simulink model "Discret_algemeine_schematische"  (Simulink 7.7)
settings: Solver=ode45  StartTime=0.0  StopTime=14  RelTol=1e-3
libraries: simulink x5
settings Model: Creator=evgenov  LastModifiedBy=Алексей
settings DebuggingCC: FcnCallInpInsideContextMsg=Enable All

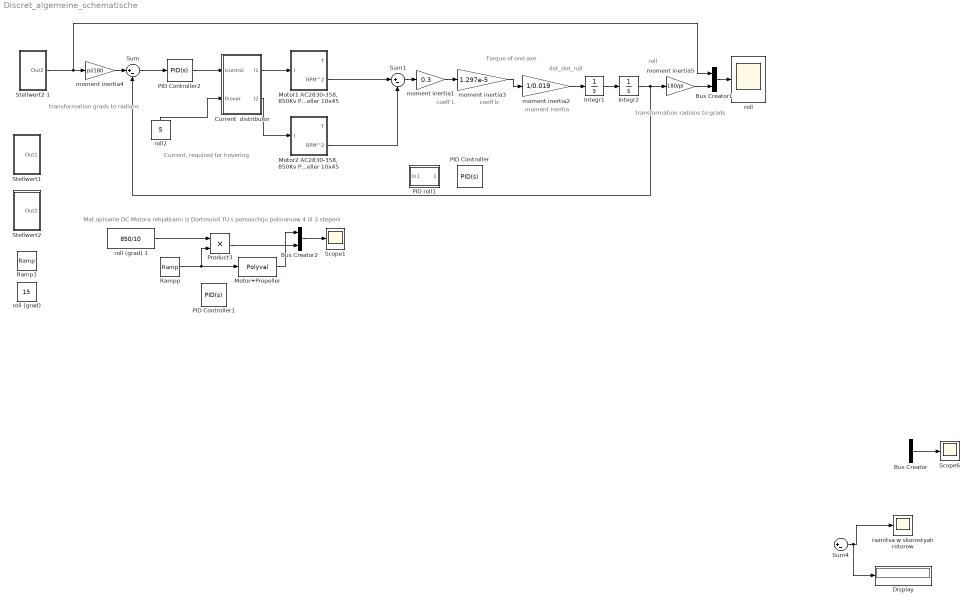
== system Discret_algemeine_schematische ==
  note: roll
  note: dot_dot_roll
  note: moment inertia
  note: Mat.opisanie DC Motora
      | rebjatkami iz Dortmund TU s pomoschiju
      | polinomow 4 ili 3 stepeni
  note: coeff L
  note: coeff b
  note: Torque of
      | one axe
  note: transformation
      | grads to radians
  note: transformation
      | radians to grads
  note: Current, required
      | for hovering
  Bus Creator : BusCreator  Inputs=2
  Bus Creator1 : BusCreator  Inputs=2
  Bus Creator2 : BusCreator  Inputs=2
  Current  distributor : Subsystem
  Display : Display
  Integr1 : Integrator
  Integr2 : Integrator
  Motor+Propeller : Polyval  Coefs="[0.0125   -0.1814   -3.6987  124.7646  -0.0000]"
  "Motor1 AC2830-358,  850Kv Propeller 10x45" : Subsystem
  "Motor2 AC2830-358,  850Kv Propeller 10x45" : Subsystem
  PID Controller : simulink/Continuous/PID Controller  SystemSampleTime=-1  Controller=PID  TimeDomain=Continuous-time  SampleTime=1  IntegratorMethod=Forward Euler  FilterMethod=Forward Euler  Form=Parallel  P=100  I=0  D=100  N=100  InitialConditionSource=internal  InitialConditionForIntegrator=0  InitialConditionForFilter=0  ExternalReset=none  LimitOutput=off  UpperSaturationLimit=0  LowerSaturationLimit=10  LinearizeAsGain=off  AntiWindupMode=back-calculation  Kb=1  TrackingMode=off  Kt=1  PParamMin=[]  PParamMax=[]  IParamMin=[]  IParamMax=[]  DParamMin=[]  DParamMax=[]  NParamMin=[]  NParamMax=[]  KbParamMin=[]  KbParamMax=[]  KtParamMin=[]  KtParamMax=[]  POutMin=[]  POutMax=[]  IOutMin=[]  IOutMax=[]  DOutMin=[]  DOutMax=[]  NOutMin=[]  NOutMax=[]  KbOutMin=[]  KbOutMax=[]  KtOutMin=[]  KtOutMax=[]  IntegratorOutMin=[]  IntegratorOutMax=[]  FilterOutMin=[]  FilterOutMax=[]  SumOutMin=[]  SumOutMax=[]  SumI1OutMin=[]  SumI1OutMax=[]  SumI2OutMin=[]  SumI2OutMax=[]  SumI3OutMin=[]  SumI3OutMax=[]  SumDOutMin=[]  SumDOutMax=[]  SaturationOutMin=[]  SaturationOutMax=[]  IntegratorContinuousStateAttributes=''  IntegratorStateMustResolveToSignalObject=off  IntegratorRTWStateStorageClass=Auto  FilterContinuousStateAttributes=''  FilterStateMustResolveToSignalObject=off  FilterRTWStateStorageClass=Auto
  PID Controller1 : simulink/Continuous/PID Controller  SystemSampleTime=-1  Controller=PID  TimeDomain=Continuous-time  SampleTime=1  IntegratorMethod=Forward Euler  FilterMethod=Forward Euler  Form=Parallel  P=0  I=0.201330059288448  D=0  N=100  InitialConditionSource=internal  InitialConditionForIntegrator=0  InitialConditionForFilter=0  ExternalReset=none  LimitOutput=off  UpperSaturationLimit=0  LowerSaturationLimit=10  LinearizeAsGain=off  AntiWindupMode=back-calculation  Kb=1  TrackingMode=off  Kt=1  PParamMin=[]  PParamMax=[]  IParamMin=[]  IParamMax=[]  DParamMin=[]  DParamMax=[]  NParamMin=[]  NParamMax=[]  KbParamMin=[]  KbParamMax=[]  KtParamMin=[]  KtParamMax=[]  POutMin=[]  POutMax=[]  IOutMin=[]  IOutMax=[]  DOutMin=[]  DOutMax=[]  NOutMin=[]  NOutMax=[]  KbOutMin=[]  KbOutMax=[]  KtOutMin=[]  KtOutMax=[]  IntegratorOutMin=[]  IntegratorOutMax=[]  FilterOutMin=[]  FilterOutMax=[]  SumOutMin=[]  SumOutMax=[]  SumI1OutMin=[]  SumI1OutMax=[]  SumI2OutMin=[]  SumI2OutMax=[]  SumI3OutMin=[]  SumI3OutMax=[]  SumDOutMin=[]  SumDOutMax=[]  SaturationOutMin=[]  SaturationOutMax=[]  IntegratorContinuousStateAttributes=''  IntegratorStateMustResolveToSignalObject=off  IntegratorRTWStateStorageClass=Auto  FilterContinuousStateAttributes=''  FilterStateMustResolveToSignalObject=off  FilterRTWStateStorageClass=Auto
  PID Controller2 : simulink/Continuous/PID Controller  SystemSampleTime=-1  Controller=PID  TimeDomain=Continuous-time  SampleTime=1  IntegratorMethod=Forward Euler  FilterMethod=Forward Euler  Form=Parallel  P=1.61212591458776e-006  I=5.412028694951e-008  D=1.06698619191158e-005  N=657.62885892053  InitialConditionSource=internal  InitialConditionForIntegrator=0  InitialConditionForFilter=0  ExternalReset=none  LimitOutput=off  UpperSaturationLimit=0  LowerSaturationLimit=10  LinearizeAsGain=off  AntiWindupMode=back-calculation  Kb=1  TrackingMode=off  Kt=1  PParamMin=[]  PParamMax=[]  IParamMin=[]  IParamMax=[]  DParamMin=[]  DParamMax=[]  NParamMin=[]  NParamMax=[]  KbParamMin=[]  KbParamMax=[]  KtParamMin=[]  KtParamMax=[]  POutMin=[]  POutMax=[]  IOutMin=[]  IOutMax=[]  DOutMin=[]  DOutMax=[]  NOutMin=[]  NOutMax=[]  KbOutMin=[]  KbOutMax=[]  KtOutMin=[]  KtOutMax=[]  IntegratorOutMin=[]  IntegratorOutMax=[]  FilterOutMin=[]  FilterOutMax=[]  SumOutMin=[]  SumOutMax=[]  SumI1OutMin=[]  SumI1OutMax=[]  SumI2OutMin=[]  SumI2OutMax=[]  SumI3OutMin=[]  SumI3OutMax=[]  SumDOutMin=[]  SumDOutMax=[]  SaturationOutMin=[]  SaturationOutMax=[]  IntegratorContinuousStateAttributes=''  IntegratorStateMustResolveToSignalObject=off  IntegratorRTWStateStorageClass=Auto  FilterContinuousStateAttributes=''  FilterStateMustResolveToSignalObject=off  FilterRTWStateStorageClass=Auto
  PID roll1 : Subsystem
  Product3 : Product  RndMeth=Zero
  Ramp1 : simulink/Sources/Ramp  SystemSampleTime=-1  slope=1  start=0  X0=0
  Rampp : simulink/Sources/Ramp  SystemSampleTime=-1  slope=1  start=0  X0=0
  Scope1 : Scope
  Scope6 : Scope
      settings: TimeRange=100  SaveName=ScopeData4
  Stellwert1 : Subsystem
  "Stellwert2 " : Subsystem
  Stellwert2 1 : Subsystem
  Sum : Sum  Inputs=|+-
  Sum1 : Sum  Inputs=|+-
  Sum4 : Sum  Inputs=|+-
  moment inertia1 : Gain  Gain=0.3
  moment inertia2 : Gain  Gain=1/0.019
  moment inertia3 : Gain  Gain=1.297e-5
  moment inertia4 : Gain  Gain=pi/180
  moment inertia5 : Gain  Gain=180/pi
  raznitsa w skorostyah rotorow : Scope
      settings: TimeRange=100  SaveName=ScopeData5
  roll : Scope
      settings: TickLabels=on  TimeRange=150  YMin=0  YMax=20
  "roll (grad) " : Constant  Value=15
  roll (grad) 1 : Constant  Value=850/10
  roll2 : Constant  Value=5
  wires:
  moment inertia4/1 -> Sum/1
  Integr2/1 -> Sum/2, moment inertia5/1
  moment inertia2/1 -> Integr1/1
  Rampp/1 -> Product3/2, Motor+Propeller/1
  Motor+Propeller/1 -> Bus Creator2/1
  Bus Creator/1 -> Scope6/1
  Sum4/1 -> Display/1, raznitsa w skorostyah rotorow/1
  Current  distributor/1(I1) -> "Motor1 AC2830-358,  850Kv Propeller 10x45"/1(I)
  Current  distributor/2(I2) -> "Motor2 AC2830-358,  850Kv Propeller 10x45"/1(I)
  moment inertia3/1 -> moment inertia2/1
  moment inertia1/1 -> moment inertia3/1
  Sum1/1 -> moment inertia1/1
  Stellwert2 1/1(Out2) -> moment inertia4/1, Bus Creator1/1
  Integr1/1 -> Integr2/1
  moment inertia5/1 -> Bus Creator1/2
  Bus Creator1/1 -> roll/1
  roll2/1 -> Current  distributor/2(Ihover)
  roll (grad) 1/1 -> Product3/1
  Bus Creator2/1 -> Scope1/1
  Product3/1 -> Bus Creator2/2
  "Motor1 AC2830-358,  850Kv Propeller 10x45"/2(RPM^2) -> Sum1/1
  "Motor2 AC2830-358,  850Kv Propeller 10x45"/2(RPM^2) -> Sum1/2
  Sum/1 -> PID Controller2/1
  PID Controller2/1 -> Current  distributor/1("Icontrol ")

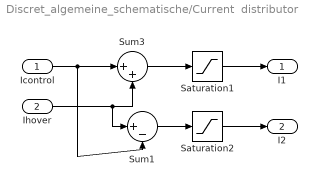
== system Discret_algemeine_schematische/Current  distributor ==
  "Icontrol " : Inport
  Ihover : Inport  Port=2
  Saturation1 : Saturate  UpperLimit=13.3  LowerLimit=0.45  ZeroCross=off
  Saturation2 : Saturate  UpperLimit=13.3  LowerLimit=0.45  ZeroCross=off
  Sum1 : Sum  Inputs=|+-
  Sum3 : Sum  Inputs=|++
  I1 : Outport
  I2 : Outport  Port=2
  wires:
  Ihover/1 -> Sum1/1, Sum3/2
  "Icontrol "/1 -> Sum3/1, Sum1/2
  Sum3/1 -> Saturation1/1
  Sum1/1 -> Saturation2/1
  Saturation2/1 -> I2/1
  Saturation1/1 -> I1/1

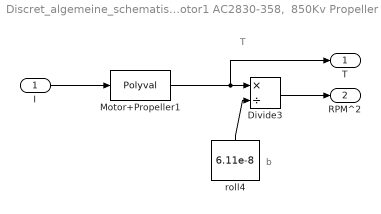
== system Discret_algemeine_schematische/Motor1 AC2830-358,  850Kv Propeller 10x45 ==
  note: b
  note: T
  I : Inport
  Divide3 : Product  Inputs=*/
  Motor+Propeller1 : Polyval  Coefs="[0.0125   -0.1814   -3.6987  124.7646  -0.0000]"
  roll4 : Constant  Value=6.11e-8
  T : Outport
  RPM^2 : Outport  Port=2
  wires:
  Divide3/1 -> RPM^2/1
  roll4/1 -> Divide3/2
  Motor+Propeller1/1 -> Divide3/1, T/1
  I/1 -> Motor+Propeller1/1

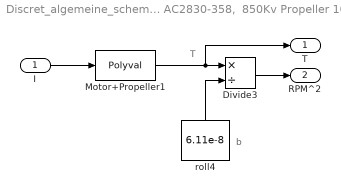
== system Discret_algemeine_schematische/Motor2 AC2830-358,  850Kv Propeller 10x45 ==
  note: T
  note: b
  I : Inport
  Divide3 : Product  Inputs=*/
  Motor+Propeller1 : Polyval  Coefs="[0.0125   -0.1814   -3.6987  124.7646  -0.0000]"
  roll4 : Constant  Value=6.11e-8
  T : Outport
  RPM^2 : Outport  Port=2
  wires:
  roll4/1 -> Divide3/2
  Divide3/1 -> RPM^2/1
  Motor+Propeller1/1 -> T/1, Divide3/1
  I/1 -> Motor+Propeller1/1

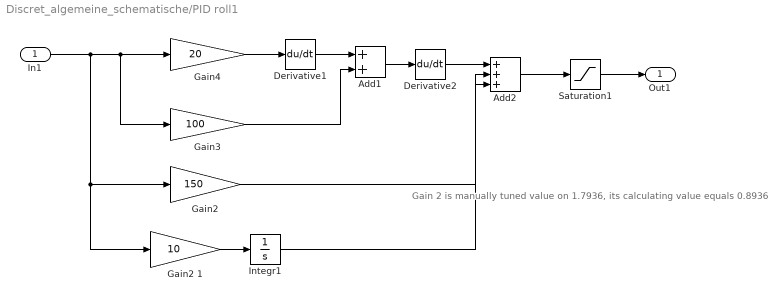
== system Discret_algemeine_schematische/PID roll1 ==
  note: Gain 2 is manually
      | tuned value on 1.7936,
      | its calculating value
      | equals 0.8936
  In1 : Inport
  Add1 : Sum
  Add2 : Sum  Inputs=+++
  Derivative1 : Derivative
  Derivative2 : Derivative
  "Gain2 " : Gain  Gain=150
  Gain2 1 : Gain  Gain=10
  Gain3 : Gain  Gain=100
  Gain4 : Gain  Gain=20
  Integr1 : Integrator
  Saturation1 : Saturate  UpperLimit=20  LowerLimit=-20  ZeroCross=off
  Out1 : Outport
  wires:
  Integr1/1 -> Add2/3
  Gain2 1/1 -> Integr1/1
  Derivative1/1 -> Add1/1
  In1/1 -> Gain2 1/1, "Gain2 "/1, Gain4/1, Gain3/1
  Gain4/1 -> Derivative1/1
  Add1/1 -> Derivative2/1
  "Gain2 "/1 -> Add2/2
  Gain3/1 -> Add1/2
  Derivative2/1 -> Add2/1
  Add2/1 -> Saturation1/1
  Saturation1/1 -> Out1/1

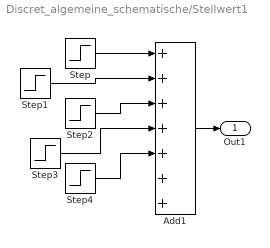
== system Discret_algemeine_schematische/Stellwert1 ==
  Add1 : Sum  Inputs=+++++++
  Step : Step  Time=0  After=5  SampleTime=0
  Step1 : Step  Time=4  After=10  SampleTime=0
  Step2 : Step  Time=9  After=30  SampleTime=0
  Step3 : Step  Time=20  After=-40  SampleTime=0
  Step4 : Step  Time=30  After=-10  SampleTime=0
  Out1 : Outport
  wires:
  ? -> Add1/7
  ? -> Add1/6
  Add1/1 -> Out1/1
  Step4/1 -> Add1/5
  Step3/1 -> Add1/4
  Step2/1 -> Add1/3
  Step1/1 -> Add1/2
  Step/1 -> Add1/1

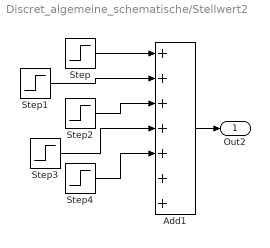
== system Discret_algemeine_schematische/Stellwert2  ==
  Add1 : Sum  Inputs=+++++++
  Step : Step  Time=0  After=5  SampleTime=0
  Step1 : Step  Time=4  After=-5  SampleTime=0
  Step2 : Step  Time=9  After=-10  SampleTime=0
  Step3 : Step  Time=20  After=-10  SampleTime=0
  Step4 : Step  Time=30  After=-10  SampleTime=0
  Out2 : Outport
  wires:
  ? -> Add1/7
  ? -> Add1/6
  Add1/1 -> Out2/1
  Step4/1 -> Add1/5
  Step3/1 -> Add1/4
  Step2/1 -> Add1/3
  Step1/1 -> Add1/2
  Step/1 -> Add1/1

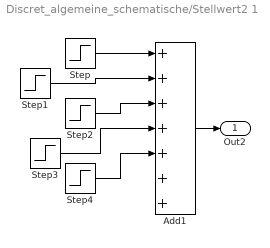
== system Discret_algemeine_schematische/Stellwert2 1 ==
  Add1 : Sum  Inputs=+++++++
  Step : Step  Time=0  After=5  SampleTime=0
  Step1 : Step  Time=4  After=-5  SampleTime=0
  Step2 : Step  Time=9  After=-10  SampleTime=0
  Step3 : Step  Time=20  After=-10  SampleTime=0
  Step4 : Step  Time=30  After=-10  SampleTime=0
  Out2 : Outport
  wires:
  Step/1 -> Add1/1
  Step1/1 -> Add1/2
  Step2/1 -> Add1/3
  Step3/1 -> Add1/4
  Step4/1 -> Add1/5
  Add1/1 -> Out2/1
  ? -> Add1/6
  ? -> Add1/7
